simulink model "continuous_model"  (R2020b)
settings: Solver=VariableStepAuto  StartTime=0.0  StopTime=20.0  RelTol=1e-3
undefined symbols (not defined in the file or in its folder): b, b_c, g, l, M, m
settings Model: Creator=kpass  LastModifiedBy=kpass

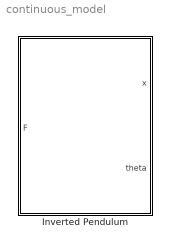
== system continuous_model ==
  Inverted Pendulum : Subsystem

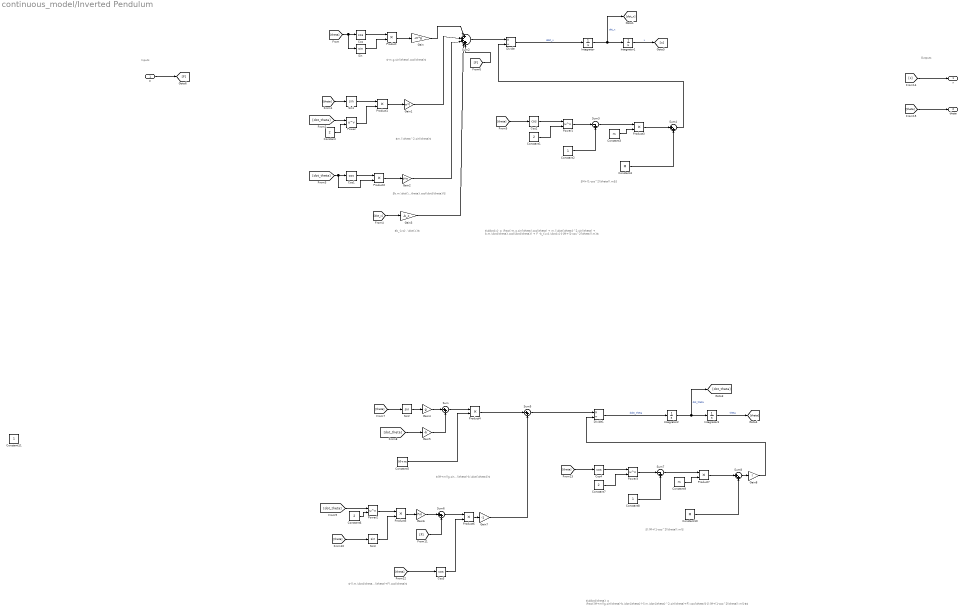
== system continuous_model/Inverted Pendulum ==
  note: Outputs
  note: Inputs
  note: $-(l.m.\dot{\theta}^2.sin(\theta)+F).cos(\theta)$
  note: $(M+m)(g.sin(\theta)-b.\dot{\theta})$
  note: $\ddot{x} = \frac{-m.g.sin(\theta).cos(\theta) + m.l.\dot{\theta}^2.sin(\theta) + b.m.\dot{\theta}.cos(\dot{\theta}) + F -b_{vz}.\dot{x}}{M+(1-cos^2(\theta)).m}$
  note: $M+(1-cos^2(\theta)).m$$
  note: $b_{vz}. \dot{x}$
  note: $b.m.\dot{\theta}.cos(\dot{\theta})$
  note: $m.l.\theta^2.sin(\theta)$
  note: $-m.g.sin(\theta).cos(\theta)$
  note: $l.(M+(1-cos^2(\theta)).m)$
  note: $\ddot{\theta} = \frac{(M+m)(g.sin(\theta)-b.\dot{\theta})-(l.m.\dot{\theta}^2.sin(\theta)+F).cos(\theta)}{l.(M+(1-cos^2(\theta)).m)}$$
  F : Inport
  Constant{,1,6..7} (4 alike) : Constant  Value=2
  Constant10 : Constant  Value=M
  Constant11 : Constant
  Constant2 : Constant
  Constant3 : Constant  Value=m
  Constant4 : Constant  Value=M
  Constant5 : Constant  Value=M+m
  Constant8 : Constant
  Constant9 : Constant  Value=m
  Cos{,1..4} (5 alike) : Trigonometry  Operator=cos
  Divide : Product  Inputs=*/
  Divide1 : Product  Inputs=*/
  Gain : Gain  Gain=-m*g
  Gain1 : Gain  Gain=m*l
  Gain2 : Gain  Gain=b*m
  Gain3 : Gain  Gain=-b_c
  Gain4 : Gain  Gain=g
  Gain5 : Gain  Gain=-b
  Gain6 : Gain  Gain=l*m
  Gain7 : Gain  Gain=-1
  Gain8 : Gain  Gain=l
  Integrator{,1..3} (4 alike) : Integrator
  Power{,1..3} (4 alike) : Math  Operator=pow  SaturateOnIntegerOverflow=on
  Product{,1..7} (8 alike) : Product
  Sin{,1..3} (4 alike) : Trigonometry
  Sum{,4..6,8} (5 alike) : Sum  Inputs=|++
  Sum2 : Sum  Inputs=|+++++
  Sum3 : Sum  Inputs=|-+
  Sum7 : Sum  Inputs=|-+
  x : Outport
  theta : Outport  Port=2
  wires:
  Product1/1 -> Gain1/1
  Power2/1 -> Product5/1
  Product/1 -> Gain/1
  Constant1/1 -> Power1/2
  Power/1 -> Product1/2
  Sum7/1 -> Product7/1
  Constant2/1 -> Sum3/2
  Gain7/1 -> Sum5/2
  Sum8/1 -> Gain8/1
  [dot_theta] -> Product2/2, Cos1/1
  [theta] -> Cos3/1
  Integrator1/1 -> [x]  "x"
  Constant3/1 -> Product3/2
  Sum3/1 -> Product3/1
  Sin/1 -> Product/2
  Cos3/1 -> Product6/2
  Constant9/1 -> Product7/2
  Integrator/1 -> [dot_x], Integrator1/1  "dot_x"
  Gain5/1 -> Sum/2
  [theta] -> Sin1/1
  Product6/1 -> Gain7/1
  Integrator3/1 -> [theta]  "theta"
  [theta] -> Cos4/1
  Gain8/1 -> Divide1/2
  Sin3/1 -> Product5/2
  Constant6/1 -> Power2/2
  [dot_x] -> Gain3/1
  Gain1/1 -> Sum2/2
  [F] -> Sum6/2
  Sin1/1 -> Product1/1
  Gain6/1 -> Sum6/1
  Product2/1 -> Gain2/1
  Cos/1 -> Product/1
  Integrator2/1 -> [dot_theta], Integrator3/1  "dot_theta"
  [theta] -> Sin/1, Cos/1
  Cos4/1 -> Power3/1
  [theta] -> theta/1
  Sum2/1 -> Divide/1
  [dot_theta] -> Gain5/1
  Sin2/1 -> Gain4/1
  Gain4/1 -> Sum/1
  Constant5/1 -> Product4/2
  Constant/1 -> Power/2
  Cos2/1 -> Power1/1
  Sum4/1 -> Divide/2
  Sum5/1 -> Divide1/1
  Cos1/1 -> Product2/1
  [dot_theta] -> Power/1
  Gain/1 -> Sum2/1
  [theta] -> Sin2/1
  [theta] -> Sin3/1
  [F] -> Sum2/5
  Divide/1 -> Integrator/1  "ddot_x"
  [x] -> x/1
  Gain2/1 -> Sum2/3
  Constant8/1 -> Sum7/2
  Divide1/1 -> Integrator2/1  "ddot_theta"
  Gain3/1 -> Sum2/4
  [theta] -> Cos2/1
  Constant4/1 -> Sum4/2
  Power1/1 -> Sum3/1
  F/1 -> [F]
  Product3/1 -> Sum4/1
  Power3/1 -> Sum7/1
  [dot_theta] -> Power2/1
  Sum/1 -> Product4/1
  Product5/1 -> Gain6/1
  Sum6/1 -> Product6/1
  Constant10/1 -> Sum8/2
  Product7/1 -> Sum8/1
  Constant7/1 -> Power3/2
  Product4/1 -> Sum5/1
